simulink model "EKF_OPT"  (R2024b)
settings: Solver=FixedStepAuto  StartTime=0.0  StopTime=250  FixedStep=0.05  RelTol=1e-3
values from neighbouring files (symbols this model uses):
  D = diag(dvec)    [singleRun.m]
undefined symbols (not defined in the file or in its folder): DiscIntNeverNeededParam, IRED, mRED, P_ic, x_ic, x_rel
libraries: slpidlib x6, simulink x2
(part 1 of 2)
settings Model: Creator=ryang  LastModifiedBy=ryang

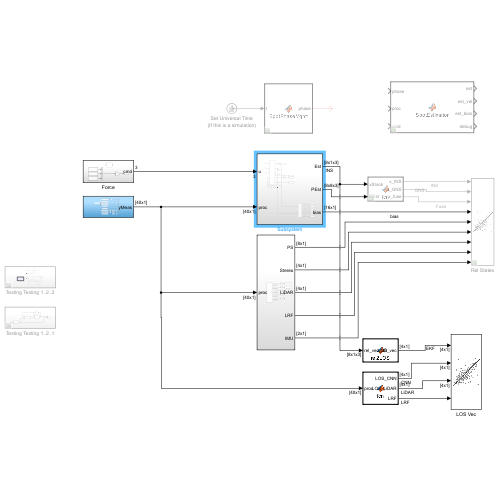
[thumbnail: Simulink's stored preview of the top-level diagram]
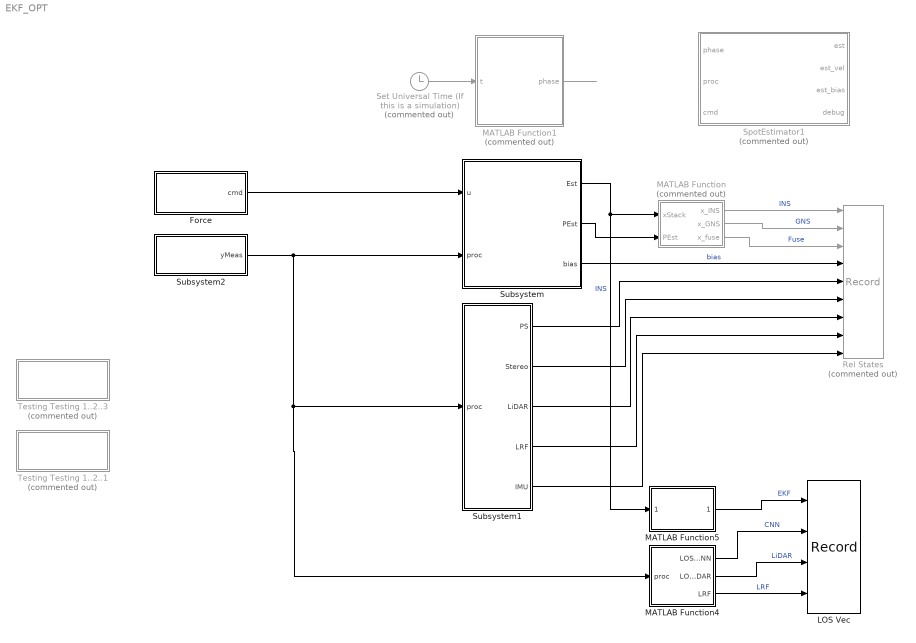
== system EKF_OPT ==
  Force : Subsystem
  LOS Vec : Record  FileSettingsInternal="{\"entries\":[{\"content\":{\"excelSettings\":{\"content\":{},\"type\":\"Streamout.ExcelSettings\"}},\"type\":\"Streamout.FileSettingStorage\",\"uuid\":\"\"}],\"packageUris\":[\"http:\\/\\/schema.mathworks.com\\/mf0\\/streamout_blocks\\/R2020a\"],\"version\":\"1.0\"}"  Layout=[2 2]  SignalsInternal="{\"entries\":[{\"content\":{\"signals\":[{\"content\":{\"blockPath\":[],\"dimensions\":[4,1],\"domain\":\"\",\"hasChildren\":true,\"lineColor\":\"#edb120\",\"lineWidth\":2,\"port\":1,\"sid\":[\"\"],\"signalID\":1,\"signalName\":\"EKF\"},\"type\":\"RecordBlkView.Signal\",\"uuid\":\"\"},{\"content\":{\"blockPath\":[],\"channel\":[1,1],\"dimensions\":[4,1],\"domain\":\"\",\"lineColor\":\"#139fff\",\"lineWidth\":2,\"parentID\":1,\"plots\":[ 1 ],\"port\":1,\"sid\":[\"\"],\"signalID\":2,\"signalName\":\"EKF\"},\"type\":\"RecordBlkView.Signal\",\"uuid\":\"\"},{\"content\":{\"blockPath\":[],\"dimensions\":[4,1],\"domain\":\"\",\"hasChildren\":true,\"lineColor\":\"#77ac30\",\"lineWidth\":2,\"port\":2,\"sid\":[\"\"],\"signalID\":3,\"signalName\":\"CNN\"},\"type\":\"RecordBlkView.Signal\",\"uuid\":\"\"},{\"content\":{\"blockPath\":[],\"channel\":[1,1],\"dimensions\":[4,1],\"domain\":\"\",\"lineColor\":\"#b746ff\",\"lineWidth\":2,\"parentID\":3,\"plots\":[ 1 ],\"port\":2,\"sid\":[\"\"],\"signalID\":4,\"signalName\":\"CNN\"},\"type\":\"RecordBlkView.Signal\",\"uuid\":\"\"},{\"content\":{\"blockPath\":[],\"dimensions\":[4,1],\"domain\":\"\",\"hasChildren\":true,\"lineColor\":\"#a2142f\",\"lineWidth\":2,\"port\":3,\"sid\":[\"\"],\"signalID\":5,\"signalName\":\"LiDAR\"},\"type\":\"RecordBlkView.Signal\",\"uuid\":\"\"},{\"content\":{\"blockPath\":[],\"channel\":[1,1],\"dimensions\":[4,1],\"domain\":\"\",\"lineColor\":\"#ff13a6\",\"lineWidth\":2,\"parentID\":5,\"plots\":[ 1 ],\"port\":3,\"sid\":[\"\"],\"signalID\":6,\"signalName\":\"LiDAR\"},\"type\":\"RecordBlkView.Signal\",\"uuid\":\"\"},{\"content\":{\"blockPath\":[],\"dimensions\":[1],\"domain\":\"\",\"lineColor\":\"#4dbeee\",\"lineWidth\":2,\"port\":4,\"sid\":[\"\"],\"signalID\":7,\"signalName\":\"LRF\"},\"type\":\"RecordBlkView.Signal\",\"uuid\":\"\"},{\"content\":{\"blockPath\":[],\"channel\":[2,1],\"dimensions\":[4,1],\"domain\":\"\",\"lineColor\":\"#fe330a\",\"lineWidth\":2,\"parentID\":1,\"plots\":[ 9 ],\"port\":1,\"sid\":[\"\"],\"signalID\":8,\"signalName\":\"EKF\"},\"type\":\"RecordBlkView.Signal\",\"uuid\":\"\"},{\"content\":{\"blockPath\":[],\"channel\":[3,1],\"dimensions\":[4,1],\"domain\":\"\",\"lineColor\":\"#22b573\",\"lineWidth\":2,\"parentID\":1,\"plots\":[ 2 ],\"port\":1,\"sid\":[\"\"],\"signalID\":9,\"signalName\":\"EKF\"},\"type\":\"RecordBlkView.Signal\",\"uuid\":\"\"},{\"content\":{\"blockPath\":[],\"channel\":[4,1],\"dimensions\":[4,1],\"domain\":\"\",\"lineColor\":\"#0072bd\",\"lineWidth\":2,\"parentID\":1,\"port\":1,\"sid\":[\"\"],\"signalID\":10,\"signalName\":\"EKF\"},\"type\":\"RecordBlkView.Signal\",\"uuid\":\"\"},{\"content\":{\"blockPath\":[],\"channel\":[2,1],\"dimensions\":[4,1],\"domain\":\"\",\"lineColor\":\"#d95319\",\"lineWidth\":2,\"parentID\":3,\"port\":2,\"sid\":[\"\"],\"signalID\":11,\"signalName\":\"CNN\"},\"type\":\"RecordBlkView.Signal\",\"uuid\":\"\"},{\"content\":{\"blockPath\":[],\"channel\":[3,1],\"dimensions\":[4,1],\"domain\":\"\",\"lineColor\":\"#edb120\",\"lineWidth\":2,\"parentID\":3,\"plots\":[ 2 ],\"port\":2,\"sid\":[\"\"],\"signalID\":12,\"signalName\":\"CNN\"},\"type\":\"RecordBlkView.Signal\",\"uuid\":\"\"},{\"content\":{\"blockPath\":[],\"channel\":[4,1],\"dimensions\":[4,1],\"domain\":\"\",\"lineColor\":\"#7e2f8e\",\"lineWidth\":2,\"parentID\":3,\"port\":2,\"sid\":[\"\"],\"signalID\":13,\"signalName\":\"CNN\"},\"type\":\"RecordBlkView.Signal\",\"uuid\":\"\"},{\"content\":{\"blockPath\":[],\"channel\":[2,1],\"dimensions\":[4,1],\"domain\":\"\",\"lineColor\":\"#77ac30\",\"lineWidth\":2,\"parentID\":5,\"plots\":[ 9 ],\"port\":3,\"sid\":[\"\"],\"signalID\":14,\"signalName\":\"LiDAR\"},\"type\":\"RecordBlkView.Signal\",\"uuid\":\"\"},{\"content\":{\"blockPath\":[],\"channel\":[3,1],\"dimensions\":[4,1],\"domain\":\"\",\"lineColor\":\"#4dbeee\",\"lineWidth\":2,\"parentID\":5,\"plots\":[ 2 ],\"port\":3,\"sid\":[\"\"],\"signalID\":15,\"signalName\":\"LiDAR\"},\"type\":\"RecordBlkView.Signal\",\"uuid\":\"\"},{\"content\":{\"blockPath\":[],\"channel\":[4,1],\"dimensions\":[4,1],\"domain\":\"\",\"lineColor\":\"#a2142f\",\"lineWidth\":2,\"parentID\":5,\"port\":3,\"sid\":[\"\"],\"signalID\":16,\"signalName\":\"LiDAR\"},\"type\":\"RecordBlkView.Signal\",\"uuid\":\"\"}]},\"type\":\"RecordBlkView.InputSignals\",\"uuid\":\"\"}],\"packageUris\":[\"http:\\/\\/schema.mathworks.com\\/mf0\\/streamout_blocks\\/R2020a\"],\"version\":\"1.0\"}"  CompatibilityTag=XY
  MATLAB Function : MATLAB Function  Commented=on  TreatAsAtomicUnit=on
  MATLAB Function1 : MATLAB Function  Commented=on  TreatAsAtomicUnit=on
  MATLAB Function4 : MATLAB Function  TreatAsAtomicUnit=on
  MATLAB Function5 : MATLAB Function  TreatAsAtomicUnit=on
  Rel States : Record  Commented=on  FileSettingsInternal="{\"entries\":[{\"content\":{\"excelSettings\":{\"content\":{},\"type\":\"Streamout.ExcelSettings\"}},\"type\":\"Streamout.FileSettingStorage\",\"uuid\":\"\"}],\"packageUris\":[\"http:\\/\\/schema.mathworks.com\\/mf0\\/streamout_blocks\\/R2020a\"],\"version\":\"1.0\"}"  Layout=[2 2]  SignalsInternal="{\"entries\":[{\"content\":{},\"type\":\"RecordBlkView.InputSignals\",\"uuid\":\"\"}],\"packageUris\":[\"http:\\/\\/schema.mathworks.com\\/mf0\\/streamout_blocks\\/R2020a\"],\"version\":\"1.0\"}"  CompatibilityTag=XY
  Set Universal Time (If this is a simulation) : Clock  Commented=on
  SpotEstimator1 : MATLAB Function  Commented=on  TreatAsAtomicUnit=on
  Subsystem : Subsystem
  Subsystem1 : Subsystem
  Subsystem2 : Subsystem
  Testing Testing 1..2..1 : Subsystem  Commented=on
  Testing Testing 1..2..3 : Subsystem  Commented=on
  wires:
  Set Universal Time (If this is a simulation)/1 -> MATLAB Function1/1(t)
  MATLAB Function1/1(phase) -> ?
  Subsystem2/1(yMeas) -> MATLAB Function4/1(proc), Subsystem1/1(proc), Subsystem/2(proc)
  MATLAB Function5/1(LOS_vec) -> LOS Vec/1  "EKF"
  MATLAB Function4/1(LOS_CNN) -> LOS Vec/2  "CNN"
  MATLAB Function4/2(LOS_LiDAR) -> LOS Vec/3  "LiDAR"
  MATLAB Function4/3(LRF) -> LOS Vec/4  "LRF"
  Subsystem/1(Est) -> MATLAB Function5/1(rel_vec_3D), MATLAB Function/1(xStack)  "INS"
  Force/1(cmd) -> Subsystem/1(u)
  MATLAB Function/1(x_INS) -> Rel States/1  "INS"
  MATLAB Function/2(x_GNS) -> Rel States/2  "GNS"
  MATLAB Function/3(x_fuse) -> Rel States/3  "Fuse"
  Subsystem/2(PEst) -> MATLAB Function/2(PEst)
  Subsystem/3(bias) -> Rel States/4  "bias"
  Subsystem1/1(PS) -> Rel States/5
  Subsystem1/2(Stereo) -> Rel States/6
  Subsystem1/3(LiDAR) -> Rel States/7
  Subsystem1/4(LRF) -> Rel States/8
  Subsystem1/5(IMU) -> Rel States/9

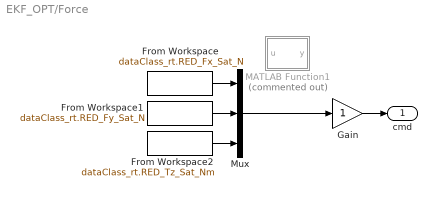
== system EKF_OPT/Force ==
  From Workspace : FromWorkspace  VariableName=dataClass_rt.RED_Fx_Sat_N
  From Workspace1 : FromWorkspace  VariableName=dataClass_rt.RED_Fy_Sat_N
  From Workspace2 : FromWorkspace  VariableName=dataClass_rt.RED_Tz_Sat_Nm
  Gain : Gain
  MATLAB Function1 : MATLAB Function  Commented=on  TreatAsAtomicUnit=on
  Mux : Mux  Inputs=3
  cmd : Outport
  wires:
  From Workspace2/1 -> Mux/3
  From Workspace1/1 -> Mux/2
  From Workspace/1 -> Mux/1
  Gain/1 -> cmd/1
  Mux/1 -> Gain/1

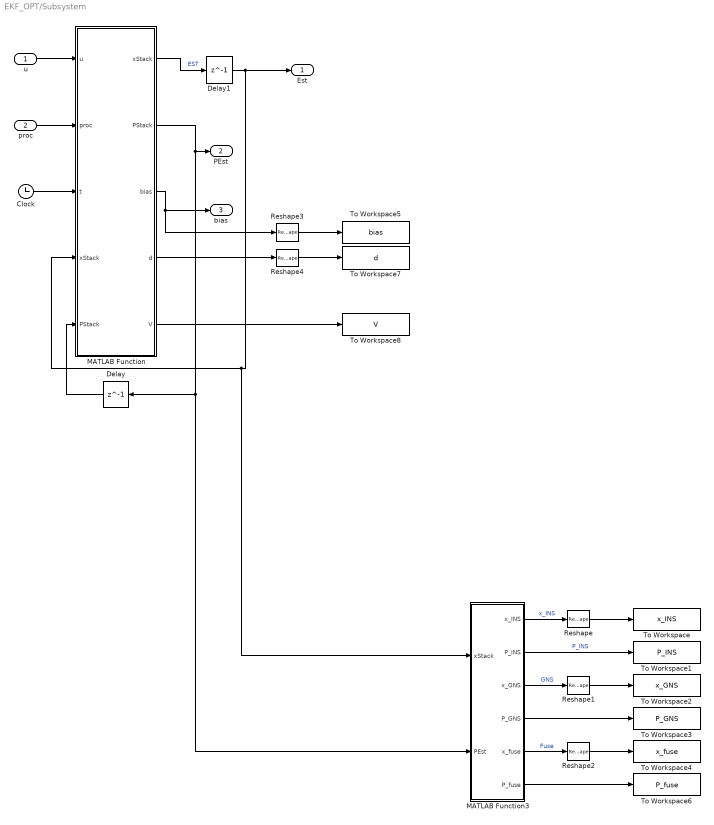
== system EKF_OPT/Subsystem ==
  u : Inport
  proc : Inport  Port=2
  Clock : Clock
  Delay : Delay  DelayLength=1  InitialCondition=P_ic
  Delay1 : Delay  DelayLength=1  InitialCondition=x_ic
  MATLAB Function : MATLAB Function  TreatAsAtomicUnit=on
  MATLAB Function3 : MATLAB Function  TreatAsAtomicUnit=on
  Reshape{,1..4} (5 alike) : Reshape  OutputDimensionality=Row vector (2-D)
  To Workspace : ToWorkspace  VariableName=x_INS  SampleTime=-1
      settings: Save2DSignal=2-D array (concatenate along first dimension)
  To Workspace1 : ToWorkspace  VariableName=P_INS  SampleTime=-1
  To Workspace2 : ToWorkspace  VariableName=x_GNS  SampleTime=-1
      settings: Save2DSignal=2-D array (concatenate along first dimension)
  To Workspace3 : ToWorkspace  VariableName=P_GNS  SampleTime=-1
  To Workspace4 : ToWorkspace  VariableName=x_fuse  SampleTime=-1
      settings: Save2DSignal=2-D array (concatenate along first dimension)
  To Workspace5 : ToWorkspace  VariableName=bias  SampleTime=-1
      settings: Save2DSignal=2-D array (concatenate along first dimension)
  To Workspace6 : ToWorkspace  VariableName=P_fuse  SampleTime=-1
  To Workspace7 : ToWorkspace  VariableName=d  SampleTime=-1
      settings: Save2DSignal=2-D array (concatenate along first dimension)
  To Workspace8 : ToWorkspace  VariableName=V  SampleTime=-1
  Est : Outport
  PEst : Outport  Port=2
  bias : Outport  Port=3
  wires:
  proc/1 -> MATLAB Function/2(proc)
  u/1 -> MATLAB Function/1(u)
  MATLAB Function/1(xStack) -> Delay1/1  "EST"
  Delay/1 -> MATLAB Function/5("PStack ")
  MATLAB Function/2(PStack) -> MATLAB Function3/2(PEst), Delay/1, PEst/1
  Delay1/1 -> MATLAB Function3/1(xStack), MATLAB Function/4("xStack "), Est/1
  MATLAB Function/3(bias) -> Reshape3/1, bias/1
  Clock/1 -> MATLAB Function/3(t)
  MATLAB Function3/2(P_INS) -> To Workspace1/1  "P_INS"
  MATLAB Function3/3(x_GNS) -> Reshape1/1  "GNS"
  MATLAB Function3/4(P_GNS) -> To Workspace3/1
  MATLAB Function3/5(x_fuse) -> Reshape2/1  "Fuse"
  MATLAB Function3/6(P_fuse) -> To Workspace6/1
  MATLAB Function3/1(x_INS) -> Reshape/1  "x_INS"
  Reshape/1 -> To Workspace/1
  Reshape1/1 -> To Workspace2/1
  Reshape2/1 -> To Workspace4/1
  Reshape3/1 -> To Workspace5/1
  MATLAB Function/4(d) -> Reshape4/1
  Reshape4/1 -> To Workspace7/1
  MATLAB Function/5(V) -> To Workspace8/1

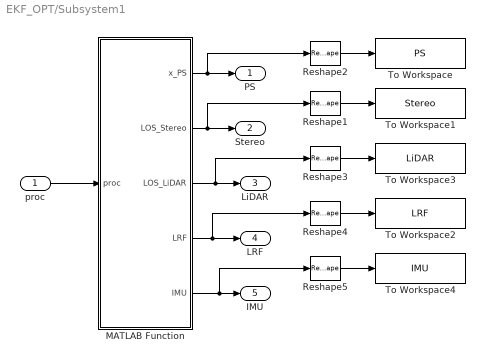
== system EKF_OPT/Subsystem1 ==
  proc : Inport
  MATLAB Function : MATLAB Function  TreatAsAtomicUnit=on
  Reshape{1..5} (5 alike) : Reshape  OutputDimensionality=Row vector (2-D)
  To Workspace : ToWorkspace  VariableName=PS  SampleTime=-1
      settings: Save2DSignal=2-D array (concatenate along first dimension)
  To Workspace1 : ToWorkspace  VariableName=Stereo  SampleTime=-1
      settings: Save2DSignal=2-D array (concatenate along first dimension)
  To Workspace2 : ToWorkspace  VariableName=LRF  SampleTime=-1
      settings: Save2DSignal=2-D array (concatenate along first dimension)
  To Workspace3 : ToWorkspace  VariableName=LiDAR  SampleTime=-1
      settings: Save2DSignal=2-D array (concatenate along first dimension)
  To Workspace4 : ToWorkspace  VariableName=IMU  SampleTime=-1
      settings: Save2DSignal=2-D array (concatenate along first dimension)
  PS : Outport
  Stereo : Outport  Port=2
  LiDAR : Outport  Port=3
  LRF : Outport  Port=4
  IMU : Outport  Port=5
  wires:
  proc/1 -> MATLAB Function/1(proc)
  MATLAB Function/1(x_PS) -> Reshape2/1, PS/1
  MATLAB Function/2(LOS_Stereo) -> Reshape1/1, Stereo/1
  MATLAB Function/3(LOS_LiDAR) -> Reshape3/1, LiDAR/1
  MATLAB Function/5(IMU) -> Reshape5/1, IMU/1
  MATLAB Function/4(LRF) -> Reshape4/1, LRF/1
  Reshape2/1 -> To Workspace/1
  Reshape1/1 -> To Workspace1/1
  Reshape3/1 -> To Workspace3/1
  Reshape4/1 -> To Workspace2/1
  Reshape5/1 -> To Workspace4/1

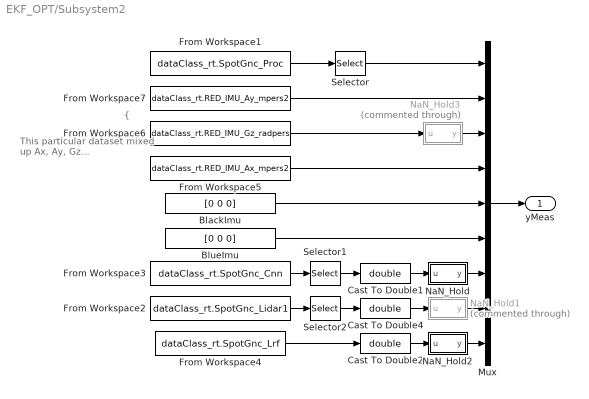
== system EKF_OPT/Subsystem2 ==
  note: {
  note: This particular dataset
      | mixed up Ax, Ay, Gz...
  BlackImu : Constant  Value=[0 0 0]
  BlueImu : Constant  Value=[0 0 0]
  Cast To Double1 : DataTypeConversion  OutDataTypeStr=double  SaturateOnIntegerOverflow=off  RndMeth=Floor
  Cast To Double2 : DataTypeConversion  OutDataTypeStr=double  SaturateOnIntegerOverflow=off  RndMeth=Floor
  Cast To Double4 : DataTypeConversion  OutDataTypeStr=double  SaturateOnIntegerOverflow=off  RndMeth=Floor
  From Workspace1 : FromWorkspace  VariableName=dataClass_rt.SpotGnc_Proc
  From Workspace2 : FromWorkspace  VariableName=dataClass_rt.SpotGnc_Lidar1
  From Workspace3 : FromWorkspace  VariableName=dataClass_rt.SpotGnc_Cnn
  From Workspace4 : FromWorkspace  VariableName=dataClass_rt.SpotGnc_Lrf
  From Workspace5 : FromWorkspace  VariableName=dataClass_rt.RED_IMU_Ax_mpers2
  From Workspace6 : FromWorkspace  VariableName=dataClass_rt.RED_IMU_Gz_radpers
  From Workspace7 : FromWorkspace  VariableName=dataClass_rt.RED_IMU_Ay_mpers2
  Mux : Mux  Inputs=9
  NaN_Hold : Subsystem
  NaN_Hold1 : Subsystem  Commented=through
  NaN_Hold2 : Subsystem
  NaN_Hold3 : Subsystem  Commented=through
  Selector : Selector  InputPortWidth=40  IndexOptions=Index vector (dialog)  Indices=[1:24]  OutputSizes=1
  Selector1 : Selector  InputPortWidth=4  IndexOptions=Index vector (dialog)  Indices=[1 2 3]  OutputSizes=1
  Selector2 : Selector  InputPortWidth=5  IndexOptions=Index vector (dialog)  Indices=[1 2 3]  OutputSizes=1
  yMeas : Outport
  wires:
  Selector/1 -> Mux/1
  Mux/1 -> yMeas/1
  From Workspace1/1 -> Selector/1
  Selector2/1 -> Cast To Double4/1
  Selector1/1 -> Cast To Double1/1
  Cast To Double1/1 -> NaN_Hold/1(u)
  From Workspace4/1 -> Cast To Double2/1
  BlackImu/1 -> Mux/5
  From Workspace2/1 -> Selector2/1
  BlueImu/1 -> Mux/6
  Cast To Double4/1 -> NaN_Hold1/1(u)
  From Workspace5/1 -> Mux/4
  From Workspace6/1 -> NaN_Hold3/1(u)
  From Workspace7/1 -> Mux/2
  Cast To Double2/1 -> NaN_Hold2/1(u)
  From Workspace3/1 -> Selector1/1
  NaN_Hold/1(y) -> Mux/7
  NaN_Hold1/1(y) -> Mux/8
  NaN_Hold2/1(y) -> Mux/9
  NaN_Hold3/1(y) -> Mux/3

== system EKF_OPT/Testing Testing 1..2..1 ==
  Clock : Clock
  Delay2 : Delay  DelayLength=1  InitialCondition=x_rel
  LQR+FeedForward : Subsystem
  MATLAB Function : MATLAB Function  TreatAsAtomicUnit=on
  MATLAB Function3 : MATLAB Function  TreatAsAtomicUnit=on
  XY Graph : Record  FileSettingsInternal="{\"entries\":[{\"content\":{\"excelSettings\":{\"content\":{},\"type\":\"Streamout.ExcelSettings\"}},\"type\":\"Streamout.FileSettingStorage\",\"uuid\":\"\"}],\"packageUris\":[\"http:\\/\\/schema.mathworks.com\\/mf0\\/streamout_blocks\\/R2020a\"],\"version\":\"1.0\"}"  Layout=[2 2]  SignalsInternal="{\"entries\":[{\"content\":{\"signals\":[{\"content\":{\"blockPath\":[],\"dimensions\":[8,1],\"domain\":\"\",\"hasChildren\":true,\"lineColor\":\"#fe330a\",\"lineWidth\":2,\"port\":1,\"signalID\":1,\"signalName\":\"true\"},\"type\":\"RecordBlkView.Signal\",\"uuid\":\"\"},{\"content\":{\"blockPath\":[],\"channel\":[1,1],\"dimensions\":[8,1],\"domain\":\"\",\"lineColor\":\"#a2142f\",\"lineWidth\":2,\"parentID\":1,\"plots\":[ 1 ],\"port\":1,\"signalID\":2,\"signalName\":\"true\"},\"type\":\"RecordBlkView.Signal\",\"uuid\":\"\"},{\"content\":{\"blockPath\":[],\"channel\":[2,1],\"dimensions\":[8,1],\"domain\":\"\",\"lineColor\":\"#0072bd\",\"lineWidth\":2,\"parentID\":1,\"plots\":[ 9 ],\"port\":1,\"signalID\":3,\"signalName\":\"true\"},\"type\":\"RecordBlkView.Signal\",\"uuid\":\"\"},{\"content\":{\"blockPath\":[],\"channel\":[3,1],\"dimensions\":[8,1],\"domain\":\"\",\"lineColor\":\"#d95319\",\"lineWidth\":2,\"parentID\":1,\"port\":1,\"signalID\":4,\"signalName\":\"true\"},\"type\":\"RecordBlkView.Signal\",\"uuid\":\"\"},{\"content\":{\"blockPath\":[],\"channel\":[4,1],\"dimensions\":[8,1],\"domain\":\"\",\"lineColor\":\"#edb120\",\"lineWidth\":2,\"parentID\":1,\"port\":1,\"signalID\":5,\"signalName\":\"true\"},\"type\":\"RecordBlkView.Signal\",\"uuid\":\"\"},{\"content\":{\"blockPath\":[],\"channel\":[5,1],\"dimensions\":[8,1],\"domain\":\"\",\"lineColor\":\"#7e2f8e\",\"lineWidth\":2,\"parentID\":1,\"port\":1,\"signalID\":6,\"signalName\":\"true\"},\"type\":\"RecordBlkView.Signal\",\"uuid\":\"\"},{\"content\":{\"blockPath\":[],\"channel\":[6,1],\"dimensions\":[8,1],\"domain\":\"\",\"lineColor\":\"#77ac30\",\"lineWidth\":2,\"parentID\":1,\"port\":1,\"signalID\":7,\"signalName\":\"true\"},\"type\":\"RecordBlkView.Signal\",\"uuid\":\"\"},{\"content\":{\"blockPath\":[],\"channel\":[7,1],\"dimensions\":[8,1],\"domain\":\"\",\"lineColor\":\"#4dbeee\",\"lineWidth\":2,\"parentID\":1,\"plots\":[ 2 ],\"port\":1,\"signalID\":8,\"signalName\":\"true\"},\"type\":\"RecordBlkView.Signal\",\"uuid\":\"\"},{\"content\":{\"blockPath\":[],\"channel\":[8,1],\"dimensions\":[8,1],\"domain\":\"\",\"lineColor\":\"#a2142f\",\"lineWidth\":2,\"parentID\":1,\"plots\":[ 10 ],\"port\":1,\"signalID\":9,\"signalName\":\"true\"},\"type\":\"RecordBlkView.Signal\",\"uuid\":\"\"},{\"content\":{\"blockPath\":[],\"dimensions\":[6,1],\"domain\":\"\",\"hasChildren\":true,\"lineColor\":\"#0072bd\",\"lineWidth\":2,\"port\":2,\"signalID\":10,\"signalName\":\"Ref\"},\"type\":\"RecordBlkView.Signal\",\"uuid\":\"\"},{\"content\":{\"blockPath\":[],\"channel\":[1,1],\"dimensions\":[6,1],\"domain\":\"\",\"lineColor\":\"#ff6929\",\"lineWidth\":2,\"parentID\":10,\"plots\":[ 1 ],\"port\":2,\"signalID\":11,\"signalName\":\"Ref\"},\"type\":\"RecordBlkView.Signal\",\"uuid\":\"\"},{\"content\":{\"blockPath\":[],\"channel\":[2,1],\"dimensions\":[6,1],\"domain\":\"\",\"lineColor\":\"#b746ff\",\"lineWidth\":2,\"parentID\":10,\"plots\":[ 9 ],\"port\":2,\"signalID\":12,\"signalName\":\"Ref\"},\"type\":\"RecordBlkView.Signal\",\"uuid\":\"\"},{\"content\":{\"blockPath\":[],\"channel\":[3,1],\"dimensions\":[6,1],\"domain\":\"\",\"lineColor\":\"#64d413\",\"lineWidth\":2,\"parentID\":10,\"plots\":[ 2 ],\"port\":2,\"signalID\":13,\"signalName\":\"Ref\"},\"type\":\"RecordBlkView.Signal\",\"uuid\":\"\"},{\"content\":{\"blockPath\":[],\"channel\":[4,1],\"dimensions\":[6,1],\"domain\":\"\",\"lineColor\":\"#ff13a6\",\"lineWidth\":2,\"parentID\":10,\"port\":2,\"signalID\":14,\"signalName\":\"Ref\"},\"type\":\"RecordBlkView.Signal\",\"uuid\":\"\"},{\"content\":{\"blockPath\":[],\"channel\":[5,1],\"dimensions\":[6,1],\"domain\":\"\",\"lineColor\":\"#fe330a\",\"lineWidth\":2,\"parentID\":10,\"port\":2,\"signalID\":15,\"signalName\":\"Ref\"},\"type\":\"RecordBlkView.Signal\",\"uuid\":\"\"},{\"content\":{\"blockPath\":[],\"channel\":[6,1],\"dimensions\":[6,1],\"domain\":\"\",\"lineColor\":\"#22b573\",\"lineWidth\":2,\"parentID\":10,\"port\":2,\"signalID\":16,\"signalName\":\"Ref\"},\"type\":\"RecordBlkView.Signal\",\"uuid\":\"\"}]},\"type\":\"RecordBlkView.InputSignals\",\"uuid\":\"\"}],\"packageUris\":[\"http:\\/\\/schema.mathworks.com\\/mf0\\/streamout_blocks\\/R2020a\"],\"version\":\"1.0\"}"  CompatibilityTag=XY
  wires:
  MATLAB Function3/1(x_new) -> XY Graph/1, Delay2/1  "true"
  Delay2/1 -> LQR+FeedForward/1(true), MATLAB Function3/1(x_old)
  MATLAB Function/1(ref_traj) -> LQR+FeedForward/2(ref_traj), XY Graph/2  "Ref"
  Clock/1 -> MATLAB Function/1(t)
  LQR+FeedForward/1(u) -> MATLAB Function3/2(u)

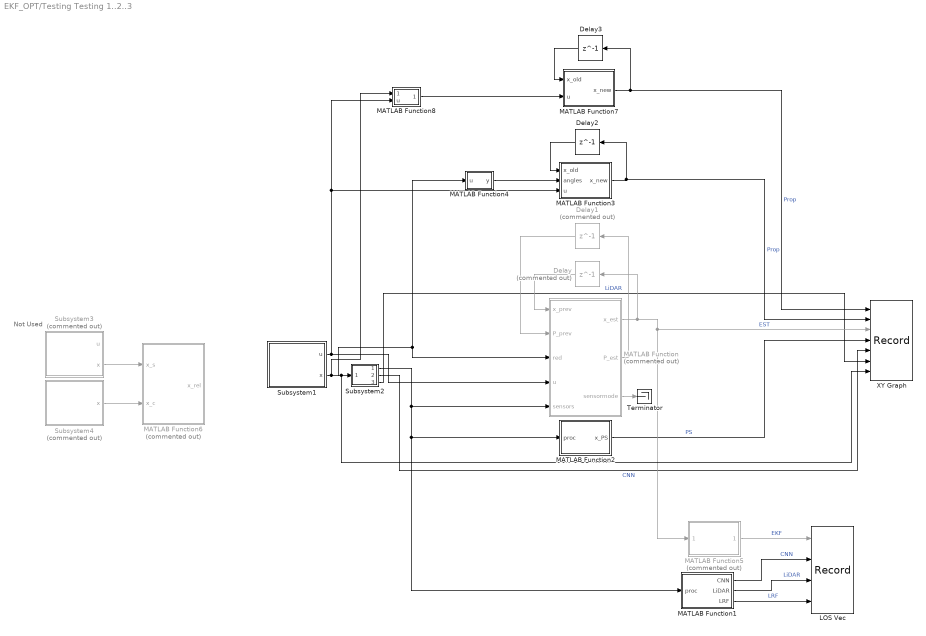
== system EKF_OPT/Testing Testing 1..2..3 ==
  note: Not Used
  Delay : Delay  Commented=on  DelayLength=1  InitialCondition=x_rel
  Delay1 : Delay  Commented=on  DelayLength=1  InitialCondition=0.2*eye(6)
  Delay2 : Delay  DelayLength=1  InitialCondition=x_rel(1:6)
  Delay3 : Delay  DelayLength=1  InitialCondition=x_rel
  LOS Vec : Record  FileSettingsInternal="{\"entries\":[{\"content\":{\"excelSettings\":{\"content\":{},\"type\":\"Streamout.ExcelSettings\"}},\"type\":\"Streamout.FileSettingStorage\",\"uuid\":\"\"}],\"packageUris\":[\"http:\\/\\/schema.mathworks.com\\/mf0\\/streamout_blocks\\/R2020a\"],\"version\":\"1.0\"}"  Layout=[1 1]  SignalsInternal="{\"entries\":[{\"content\":{},\"type\":\"RecordBlkView.InputSignals\",\"uuid\":\"\"}],\"packageUris\":[\"http:\\/\\/schema.mathworks.com\\/mf0\\/streamout_blocks\\/R2020a\"],\"version\":\"1.0\"}"  VisualizationBindings="{\"sparklinesplugin\":{\"info\":[{\"bindingParametersList\":[],\"subplotID\":1}]}}"  CompatibilityTag=XY
  MATLAB Function : MATLAB Function  Commented=on  TreatAsAtomicUnit=on
  MATLAB Function1 : MATLAB Function  TreatAsAtomicUnit=on
  MATLAB Function2 : MATLAB Function  TreatAsAtomicUnit=on
  MATLAB Function3 : MATLAB Function  TreatAsAtomicUnit=on
  MATLAB Function4 : MATLAB Function  TreatAsAtomicUnit=on
  MATLAB Function5 : MATLAB Function  Commented=on  TreatAsAtomicUnit=on
  MATLAB Function6 : MATLAB Function  Commented=on  TreatAsAtomicUnit=on
  MATLAB Function7 : MATLAB Function  TreatAsAtomicUnit=on
  MATLAB Function8 : MATLAB Function  TreatAsAtomicUnit=on
  Subsystem1 : Subsystem
  Subsystem2 : Subsystem
  Subsystem3 : Subsystem  Commented=on
  Subsystem4 : Subsystem  Commented=on
  Terminator : Terminator
  XY Graph : Record  FileSettingsInternal="{\"entries\":[{\"content\":{\"excelSettings\":{\"content\":{},\"type\":\"Streamout.ExcelSettings\"}},\"type\":\"Streamout.FileSettingStorage\",\"uuid\":\"\"}],\"packageUris\":[\"http:\\/\\/schema.mathworks.com\\/mf0\\/streamout_blocks\\/R2020a\"],\"version\":\"1.0\"}"  Layout=[2 2]  SignalsInternal="{\"entries\":[{\"content\":{},\"type\":\"RecordBlkView.InputSignals\",\"uuid\":\"\"}],\"packageUris\":[\"http:\\/\\/schema.mathworks.com\\/mf0\\/streamout_blocks\\/R2020a\"],\"version\":\"1.0\"}"  CompatibilityTag=XY
  wires:
  MATLAB Function1/1(CNN) -> LOS Vec/2  "CNN"
  Subsystem2/3(LiDAR) -> XY Graph/6  "LiDAR"
  MATLAB Function5/1(LOS_vec) -> LOS Vec/1  "EKF"
  Subsystem2/2(CNN) -> XY Graph/5  "CNN"
  MATLAB Function1/2(LiDAR) -> LOS Vec/3  "LiDAR"
  MATLAB Function2/1(x_PS) -> XY Graph/4  "PS"
  MATLAB Function/3(sensormode) -> Terminator/1
  MATLAB Function/2(P_est) -> Delay1/1
  Subsystem2/1(proc) -> MATLAB Function1/1(proc), MATLAB Function2/1(proc), MATLAB Function/5(sensors)
  Delay/1 -> MATLAB Function/1(x_prev)
  Delay1/1 -> MATLAB Function/2(P_prev)
  MATLAB Function1/3(LRF) -> LOS Vec/4  "LRF"
  MATLAB Function/1(x_est) -> Delay/1, MATLAB Function5/1(rel_vec), XY Graph/3  "EST"
  Subsystem1/1(u) -> MATLAB Function8/2(u), MATLAB Function3/3(u), MATLAB Function/4(u)
  Subsystem1/2(x) -> MATLAB Function8/1(theta), MATLAB Function4/1(u), MATLAB Function/3(red), XY Graph/7, Subsystem2/1(RED)
  MATLAB Function3/1(x_new) -> XY Graph/2, Delay2/1  "Prop"
  Delay2/1 -> MATLAB Function3/1(x_old)
  MATLAB Function4/1(y) -> MATLAB Function3/2(angles)
  Subsystem3/2(x) -> MATLAB Function6/1(x_s)
  Subsystem4/1(x) -> MATLAB Function6/2(x_c)
  MATLAB Function7/1(x_new) -> XY Graph/1, Delay3/1  "Prop"
  Delay3/1 -> MATLAB Function7/1(x_old)
  MATLAB Function8/1(u_body) -> MATLAB Function7/2(u)

== system EKF_OPT/Subsystem2/NaN_Hold ==
  u : Inport
  Delay : Delay  DelayLength=1
  MATLAB Function : MATLAB Function  TreatAsAtomicUnit=on
  y : Outport
  wires:
  u/1 -> Delay/1, MATLAB Function/1(u_curr)
  MATLAB Function/1(y) -> y/1
  Delay/1 -> MATLAB Function/2(u_prev)

== system EKF_OPT/Subsystem2/NaN_Hold1 ==
  u : Inport
  Delay : Delay  DelayLength=1
  MATLAB Function : MATLAB Function  TreatAsAtomicUnit=on
  y : Outport
  wires:
  u/1 -> Delay/1, MATLAB Function/1(u_curr)
  MATLAB Function/1(y) -> y/1
  Delay/1 -> MATLAB Function/2(u_prev)

== system EKF_OPT/Subsystem2/NaN_Hold2 ==
  u : Inport
  Delay : Delay  DelayLength=1
  MATLAB Function : MATLAB Function  TreatAsAtomicUnit=on
  y : Outport
  wires:
  u/1 -> Delay/1, MATLAB Function/1(u_curr)
  MATLAB Function/1(y) -> y/1
  Delay/1 -> MATLAB Function/2(u_prev)

== system EKF_OPT/Subsystem2/NaN_Hold3 ==
  u : Inport
  Delay : Delay  DelayLength=1
  MATLAB Function : MATLAB Function  TreatAsAtomicUnit=on
  y : Outport
  wires:
  Delay/1 -> MATLAB Function/2(u_prev)
  MATLAB Function/1(y) -> y/1
  u/1 -> MATLAB Function/1(u_curr), Delay/1

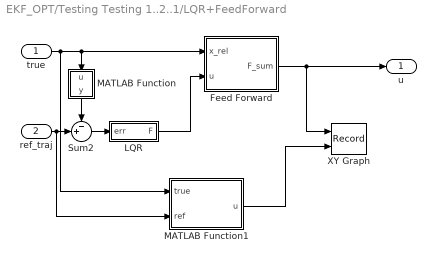
== system EKF_OPT/Testing Testing 1..2..1/LQR+FeedForward ==
  true : Inport
  ref_traj : Inport  Port=2
  Feed Forward : MATLAB Function  TreatAsAtomicUnit=on
  LQR : MATLAB Function  TreatAsAtomicUnit=on
  MATLAB Function : MATLAB Function  TreatAsAtomicUnit=on
  MATLAB Function1 : MATLAB Function  TreatAsAtomicUnit=on
  Sum2 : Sum  Inputs=-+|
  XY Graph : Record  FileSettingsInternal="{\"entries\":[{\"content\":{\"excelSettings\":{\"content\":{},\"type\":\"Streamout.ExcelSettings\"}},\"type\":\"Streamout.FileSettingStorage\",\"uuid\":\"\"}],\"packageUris\":[\"http:\\/\\/schema.mathworks.com\\/mf0\\/streamout_blocks\\/R2020a\"],\"version\":\"1.0\"}"  Layout=[1 1]  SignalsInternal="{\"entries\":[{\"content\":{\"signals\":[{\"content\":{\"blockPath\":[],\"dimensions\":[1],\"domain\":\"\",\"lineColor\":\"#a2142f\",\"plots\":[ 1 ],\"port\":1,\"signalID\":1,\"signalName\":\"XY Graph:1\"},\"type\":\"RecordBlkView.Signal\",\"uuid\":\"\"},{\"content\":{\"blockPath\":[],\"dimensions\":[1],\"domain\":\"\",\"lineColor\":\"#139fff\",\"plots\":[ 1 ],\"port\":2,\"signalID\":2,\"signalName\":\"XY Graph:2\"},\"type\":\"RecordBlkView.Signal\",\"uuid\":\"\"}]},\"type\":\"RecordBlkView.InputSignals\",\"uuid\":\"\"}],\"packageUris\":[\"http:\\/\\/schema.mathworks.com\\/mf0\\/streamout_blocks\\/R2020a\"],\"version\":\"1.0\"}"  VisualizationBindings="{\"xyplotplugin\":{\"info\":[{\"series\":[{\"bindingParametersList\":[{\"parameter\":\"X-Axis\",\"signalID\":1,\"signalName\":\"XY Graph:1\"},{\"parameter\":\"Y-Axis\",\"signalID\":2,\"signalName\":\"XY Graph:2\"}],\"seriesID\":0}],\"subplotID\":1}]}}"  CompatibilityTag=XY
  u : Outport
  wires:
  Sum2/1 -> LQR/1(err)
  true/1 -> MATLAB Function1/1(true), MATLAB Function/1(u), Feed Forward/1(x_rel)
  ref_traj/1 -> MATLAB Function1/2(ref), Sum2/2
  MATLAB Function/1(y) -> Sum2/1
  LQR/1(F) -> Feed Forward/2(u)
  Feed Forward/1(F_sum) -> XY Graph/1, u/1
  MATLAB Function1/1(u) -> XY Graph/2

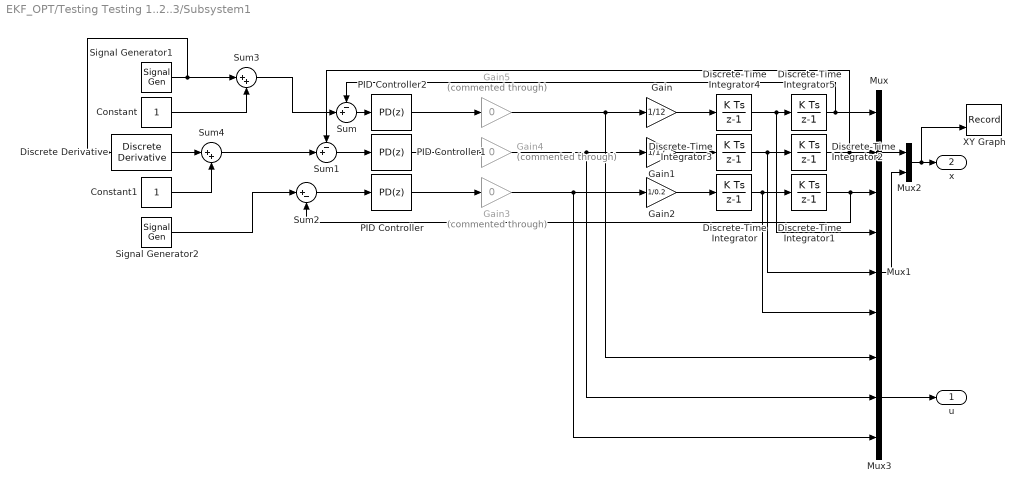
== system EKF_OPT/Testing Testing 1..2..3/Subsystem1 ==
  Constant : Constant
  Constant1 : Constant
  Discrete Derivative : simulink/Discrete/Discrete Derivative  gainval=1.0  ICPrevScaledInput=0.0  OutMin=[]  OutMax=[]  OutDataType=fixdt(1, 16)  OutScaling=2^-10  DoSatur=off
  Discrete-Time Integrator : DiscreteIntegrator  InitialCondition=-0.3  SampleTime=-1  ICPrevOutput=DiscIntNeverNeededParam  ICPrevScaledInput=DiscIntNeverNeededParam
  Discrete-Time Integrator1 : DiscreteIntegrator  SampleTime=-1  ICPrevOutput=DiscIntNeverNeededParam  ICPrevScaledInput=DiscIntNeverNeededParam
  Discrete-Time Integrator2 : DiscreteIntegrator  InitialCondition=2  SampleTime=-1  ICPrevOutput=DiscIntNeverNeededParam  ICPrevScaledInput=DiscIntNeverNeededParam
  Discrete-Time Integrator3 : DiscreteIntegrator  InitialCondition=0.2  SampleTime=-1  ICPrevOutput=DiscIntNeverNeededParam  ICPrevScaledInput=DiscIntNeverNeededParam
  Discrete-Time Integrator4 : DiscreteIntegrator  InitialCondition=-0.1  SampleTime=-1  ICPrevOutput=DiscIntNeverNeededParam  ICPrevScaledInput=DiscIntNeverNeededParam
  Discrete-Time Integrator5 : DiscreteIntegrator  InitialCondition=1  SampleTime=-1  ICPrevOutput=DiscIntNeverNeededParam  ICPrevScaledInput=DiscIntNeverNeededParam
  Gain : Gain  Gain=1/12
  Gain1 : Gain  Gain=1/12
  Gain2 : Gain  Gain=1/0.2
  Gain3 : Gain  Commented=through  Gain=0
  Gain4 : Gain  Commented=through  Gain=0
  Gain5 : Gain  Commented=through  Gain=0
  Mux : Mux  Inputs=3
  Mux1 : Mux  Inputs=3
  Mux2 : Mux  Inputs=2
  Mux3 : Mux  Inputs=3
  PID Controller : slpidlib/PID Controller  Controller=PD  Form=Parallel  TimeDomain=Discrete-time  UseExternalTs=off  SampleTime=-1  IntegratorMethod=Forward Euler  FilterMethod=Forward Euler  ControllerParametersSource=internal  P=0.00863228174020387  I=1  UseKiTs=off  D=0.441408383064275  UseExternalDerivativeSource=off  N=18.5475442531041  UseFilter=on  TunerSelectOption=Transfer Function Based (PID Tuner App)  InitialConditionSource=internal  InitialConditionForIntegrator=0  InitialConditionForFilter=0  DifferentiatorICPrevScaledInput=0  ExternalReset=none  TrackingMode=off  Kt=1  LimitOutput=off  SatLimitsSource=internal  UpperSaturationLimit=inf  LowerSaturationLimit=-inf  LinearizeAsGain=on  AntiWindupMode=none  Kb=1  LimitIntegrator=off  UpperIntegratorSaturationLimit=inf  LowerIntegratorSaturationLimit=-inf  POutMin=[]  POutMax=[]  IOutMin=[]  IOutMax=[]  DOutMin=[]  DOutMax=[]  NOutMin=[]  NOutMax=[]  SumOutMin=[]  SumOutMax=[]  SaturationOutMin=[]  SaturationOutMax=[]  PParamMin=[]  PParamMax=[]  IParamMin=[]  IParamMax=[]  DParamMin=[]  DParamMax=[]  NParamMin=[]  NParamMax=[]  KbParamMin=[]  KbParamMax=[]  KtParamMin=[]  KtParamMax=[]  KbOutMin=[]  KbOutMax=[]  KtOutMin=[]  KtOutMax=[]  IntegratorOutMin=[]  IntegratorOutMax=[]  FilterOutMin=[]  FilterOutMax=[]  SumI1OutMin=[]  SumI1OutMax=[]  SumI2OutMin=[]  SumI2OutMax=[]  SumI3OutMin=[]  SumI3OutMax=[]  SumI4OutMin=[]  SumI4OutMax=[]  SumDOutMin=[]  SumDOutMax=[]  DifferentiatorOutMin=[]  DifferentiatorOutMax=[]  FilterDiffOutCoefMin=[]  FilterDiffOutCoefMax=[]  ReciprocalOutMin=[]  ReciprocalOutMax=[]  SumDenOutMin=[]  SumDenOutMax=[]  SumNumOutMin=[]  SumNumOutMax=[]  DivideOutMin=[]  DivideOutMax=[]  UdiffTsProdOutMin=[]  UdiffTsProdOutMax=[]  NTsProdOutMin=[]  NTsProdOutMax=[]  UintegralTsProdOutMin=[]  UintegralTsProdOutMax=[]  UngainTsProdOutMin=[]  UngainTsProdOutMax=[]  ClampingZeroOutDataTypeStr=Inherit: Inherit via back propagation  ClampingZeroOutMin=[]  ClampingZeroOutMax=[]  FilterDenConstantOutDataTypeStr=Inherit: Inherit via back propagation  FilterDenConstantOutMin=[]  FilterDenConstantOutMax=[]  PCopyOutDataTypeStr=Inherit: Inherit via back propagation  PCopyOutMin=[]  PCopyOutMax=[]  NCopyOutDataTypeStr=Inherit: Inherit via back propagation  NCopyOutMin=[]  NCopyOutMax=[]  IntegratorContinuousStateAttributes=''  IntegratorStateMustResolveToSignalObject=off  IntegratorRTWStateStorageClass=Auto  FilterContinuousStateAttributes=''  FilterStateMustResolveToSignalObject=off  FilterRTWStateStorageClass=Auto  ParallelPVariant=InternalParameters  IdealPVariant=Disabled  IVariant=Disabled  DVariant=InternalParameters  IntegratorVariant=Disabled  SatVariant=Disabled  AWVariant=Disabled  PCopyVariant=Disabled  TRVariant=Disabled  FdbkBlocksVariant=Forward  IdealPFdbkVariant=Disabled  SatFdbkVariant=Disabled  DerivativeFilterVariant=ForwardEulerFilter  NVariant=InternalParameters  NCopyVariant=Disabled  FilterICVariant=InternalICsFilter  IntegratorICVariant=Disabled  ExternalResetVariant=Disabled  TRSumVariant=Passthrough  SumFdbkVariant=Disabled  SumVariant=Sum_PD  TsampFilterVariant=InternalTs  TsampNgainVariant=Passthrough  TsampIntegralVariant=Disabled_SignalSpec  ExternalSaturationOutDataTypeStr=Inherit: Same as second input  DerivativeSourceVariant=ErrorSignal  PreIntVariant=InternalPreInt
  PID Controller1 : slpidlib/PID Controller  Controller=PD  Form=Parallel  TimeDomain=Discrete-time  UseExternalTs=off  SampleTime=-1  IntegratorMethod=Forward Euler  FilterMethod=Forward Euler  ControllerParametersSource=internal  P=0.245018327394247  I=1  UseKiTs=off  D=18.2758094977982  UseExternalDerivativeSource=off  N=17.9496179817315  UseFilter=on  TunerSelectOption=Transfer Function Based (PID Tuner App)  InitialConditionSource=internal  InitialConditionForIntegrator=0  InitialConditionForFilter=0  DifferentiatorICPrevScaledInput=0  ExternalReset=none  TrackingMode=off  Kt=1  LimitOutput=off  SatLimitsSource=internal  UpperSaturationLimit=inf  LowerSaturationLimit=-inf  LinearizeAsGain=on  AntiWindupMode=none  Kb=1  LimitIntegrator=off  UpperIntegratorSaturationLimit=inf  LowerIntegratorSaturationLimit=-inf  POutMin=[]  POutMax=[]  IOutMin=[]  IOutMax=[]  DOutMin=[]  DOutMax=[]  NOutMin=[]  NOutMax=[]  SumOutMin=[]  SumOutMax=[]  SaturationOutMin=[]  SaturationOutMax=[]  PParamMin=[]  PParamMax=[]  IParamMin=[]  IParamMax=[]  DParamMin=[]  DParamMax=[]  NParamMin=[]  NParamMax=[]  KbParamMin=[]  KbParamMax=[]  KtParamMin=[]  KtParamMax=[]  KbOutMin=[]  KbOutMax=[]  KtOutMin=[]  KtOutMax=[]  IntegratorOutMin=[]  IntegratorOutMax=[]  FilterOutMin=[]  FilterOutMax=[]  SumI1OutMin=[]  SumI1OutMax=[]  SumI2OutMin=[]  SumI2OutMax=[]  SumI3OutMin=[]  SumI3OutMax=[]  SumI4OutMin=[]  SumI4OutMax=[]  SumDOutMin=[]  SumDOutMax=[]  DifferentiatorOutMin=[]  DifferentiatorOutMax=[]  FilterDiffOutCoefMin=[]  FilterDiffOutCoefMax=[]  ReciprocalOutMin=[]  ReciprocalOutMax=[]  SumDenOutMin=[]  SumDenOutMax=[]  SumNumOutMin=[]  SumNumOutMax=[]  DivideOutMin=[]  DivideOutMax=[]  UdiffTsProdOutMin=[]  UdiffTsProdOutMax=[]  NTsProdOutMin=[]  NTsProdOutMax=[]  UintegralTsProdOutMin=[]  UintegralTsProdOutMax=[]  UngainTsProdOutMin=[]  UngainTsProdOutMax=[]  ClampingZeroOutDataTypeStr=Inherit: Inherit via back propagation  ClampingZeroOutMin=[]  ClampingZeroOutMax=[]  FilterDenConstantOutDataTypeStr=Inherit: Inherit via back propagation  FilterDenConstantOutMin=[]  FilterDenConstantOutMax=[]  PCopyOutDataTypeStr=Inherit: Inherit via back propagation  PCopyOutMin=[]  PCopyOutMax=[]  NCopyOutDataTypeStr=Inherit: Inherit via back propagation  NCopyOutMin=[]  NCopyOutMax=[]  IntegratorContinuousStateAttributes=''  IntegratorStateMustResolveToSignalObject=off  IntegratorRTWStateStorageClass=Auto  FilterContinuousStateAttributes=''  FilterStateMustResolveToSignalObject=off  FilterRTWStateStorageClass=Auto  ParallelPVariant=InternalParameters  IdealPVariant=Disabled  IVariant=Disabled  DVariant=InternalParameters  IntegratorVariant=Disabled  SatVariant=Disabled  AWVariant=Disabled  PCopyVariant=Disabled  TRVariant=Disabled  FdbkBlocksVariant=Forward  IdealPFdbkVariant=Disabled  SatFdbkVariant=Disabled  DerivativeFilterVariant=ForwardEulerFilter  NVariant=InternalParameters  NCopyVariant=Disabled  FilterICVariant=InternalICsFilter  IntegratorICVariant=Disabled  ExternalResetVariant=Disabled  TRSumVariant=Passthrough  SumFdbkVariant=Disabled  SumVariant=Sum_PD  TsampFilterVariant=InternalTs  TsampNgainVariant=Passthrough  TsampIntegralVariant=Disabled_SignalSpec  ExternalSaturationOutDataTypeStr=Inherit: Same as second input  DerivativeSourceVariant=ErrorSignal  PreIntVariant=InternalPreInt
  PID Controller2 : slpidlib/PID Controller  Controller=PD  Form=Parallel  TimeDomain=Discrete-time  UseExternalTs=off  SampleTime=-1  IntegratorMethod=Forward Euler  FilterMethod=Forward Euler  ControllerParametersSource=internal  P=0.245018327394247  I=1  UseKiTs=off  D=18.2758094977982  UseExternalDerivativeSource=off  N=17.9496179817315  UseFilter=on  TunerSelectOption=Transfer Function Based (PID Tuner App)  InitialConditionSource=internal  InitialConditionForIntegrator=0  InitialConditionForFilter=0  DifferentiatorICPrevScaledInput=0  ExternalReset=none  TrackingMode=off  Kt=1  LimitOutput=off  SatLimitsSource=internal  UpperSaturationLimit=inf  LowerSaturationLimit=-inf  LinearizeAsGain=on  AntiWindupMode=none  Kb=1  LimitIntegrator=off  UpperIntegratorSaturationLimit=inf  LowerIntegratorSaturationLimit=-inf  POutMin=[]  POutMax=[]  IOutMin=[]  IOutMax=[]  DOutMin=[]  DOutMax=[]  NOutMin=[]  NOutMax=[]  SumOutMin=[]  SumOutMax=[]  SaturationOutMin=[]  SaturationOutMax=[]  PParamMin=[]  PParamMax=[]  IParamMin=[]  IParamMax=[]  DParamMin=[]  DParamMax=[]  NParamMin=[]  NParamMax=[]  KbParamMin=[]  KbParamMax=[]  KtParamMin=[]  KtParamMax=[]  KbOutMin=[]  KbOutMax=[]  KtOutMin=[]  KtOutMax=[]  IntegratorOutMin=[]  IntegratorOutMax=[]  FilterOutMin=[]  FilterOutMax=[]  SumI1OutMin=[]  SumI1OutMax=[]  SumI2OutMin=[]  SumI2OutMax=[]  SumI3OutMin=[]  SumI3OutMax=[]  SumI4OutMin=[]  SumI4OutMax=[]  SumDOutMin=[]  SumDOutMax=[]  DifferentiatorOutMin=[]  DifferentiatorOutMax=[]  FilterDiffOutCoefMin=[]  FilterDiffOutCoefMax=[]  ReciprocalOutMin=[]  ReciprocalOutMax=[]  SumDenOutMin=[]  SumDenOutMax=[]  SumNumOutMin=[]  SumNumOutMax=[]  DivideOutMin=[]  DivideOutMax=[]  UdiffTsProdOutMin=[]  UdiffTsProdOutMax=[]  NTsProdOutMin=[]  NTsProdOutMax=[]  UintegralTsProdOutMin=[]  UintegralTsProdOutMax=[]  UngainTsProdOutMin=[]  UngainTsProdOutMax=[]  ClampingZeroOutDataTypeStr=Inherit: Inherit via back propagation  ClampingZeroOutMin=[]  ClampingZeroOutMax=[]  FilterDenConstantOutDataTypeStr=Inherit: Inherit via back propagation  FilterDenConstantOutMin=[]  FilterDenConstantOutMax=[]  PCopyOutDataTypeStr=Inherit: Inherit via back propagation  PCopyOutMin=[]  PCopyOutMax=[]  NCopyOutDataTypeStr=Inherit: Inherit via back propagation  NCopyOutMin=[]  NCopyOutMax=[]  IntegratorContinuousStateAttributes=''  IntegratorStateMustResolveToSignalObject=off  IntegratorRTWStateStorageClass=Auto  FilterContinuousStateAttributes=''  FilterStateMustResolveToSignalObject=off  FilterRTWStateStorageClass=Auto  ParallelPVariant=InternalParameters  IdealPVariant=Disabled  IVariant=Disabled  DVariant=InternalParameters  IntegratorVariant=Disabled  SatVariant=Disabled  AWVariant=Disabled  PCopyVariant=Disabled  TRVariant=Disabled  FdbkBlocksVariant=Forward  IdealPFdbkVariant=Disabled  SatFdbkVariant=Disabled  DerivativeFilterVariant=ForwardEulerFilter  NVariant=InternalParameters  NCopyVariant=Disabled  FilterICVariant=InternalICsFilter  IntegratorICVariant=Disabled  ExternalResetVariant=Disabled  TRSumVariant=Passthrough  SumFdbkVariant=Disabled  SumVariant=Sum_PD  TsampFilterVariant=InternalTs  TsampNgainVariant=Passthrough  TsampIntegralVariant=Disabled_SignalSpec  ExternalSaturationOutDataTypeStr=Inherit: Same as second input  DerivativeSourceVariant=ErrorSignal  PreIntVariant=InternalPreInt
  Signal Generator1 : SignalGenerator  Frequency=2*pi/60  Units=rad/sec
  Signal Generator2 : SignalGenerator  Amplitude=0.01  Frequency=2*pi/60  Units=rad/sec
  Sum : Sum  Inputs=-+|
  Sum1 : Sum  Inputs=-+|
  Sum2 : Sum  Inputs=|+-
  Sum3 : Sum  Inputs=|++
  Sum4 : Sum  Inputs=|++
  XY Graph : Record  FileSettingsInternal="{\"entries\":[{\"content\":{\"excelSettings\":{\"content\":{},\"type\":\"Streamout.ExcelSettings\"}},\"type\":\"Streamout.FileSettingStorage\",\"uuid\":\"\"}],\"packageUris\":[\"http:\\/\\/schema.mathworks.com\\/mf0\\/streamout_blocks\\/R2020a\"],\"version\":\"1.0\"}"  Layout=[1 1]  SignalsInternal="{\"entries\":[{\"content\":{},\"type\":\"RecordBlkView.InputSignals\",\"uuid\":\"\"}],\"packageUris\":[\"http:\\/\\/schema.mathworks.com\\/mf0\\/streamout_blocks\\/R2020a\"],\"version\":\"1.0\"}"  VisualizationBindings="{\"xyplotplugin\":{\"info\":[{\"series\":[],\"subplotID\":1}]}}"  CompatibilityTag=XY
  u : Outport
  x : Outport  Port=2
  wires:
  Discrete-Time Integrator4/1 -> Discrete-Time Integrator5/1, Mux1/1
  Discrete-Time Integrator3/1 -> Discrete-Time Integrator2/1, Mux1/2
  Discrete-Time Integrator/1 -> Discrete-Time Integrator1/1, Mux1/3
  Discrete-Time Integrator1/1 -> Sum2/2, Mux/3
  Discrete-Time Integrator2/1 -> Mux/2, Sum1/1
  Discrete-Time Integrator5/1 -> Mux/1, Sum/1
  PID Controller2/1 -> Gain5/1
  PID Controller1/1 -> Gain4/1
  PID Controller/1 -> Gain3/1
  Mux/1 -> Mux2/1
  Mux1/1 -> Mux2/2
  Mux2/1 -> XY Graph/2, x/1
  Gain/1 -> Discrete-Time Integrator4/1
  Gain1/1 -> Discrete-Time Integrator3/1
  Gain2/1 -> Discrete-Time Integrator/1
  Mux3/1 -> u/1
  Sum/1 -> PID Controller2/1
  Sum2/1 -> PID Controller/1
  Sum1/1 -> PID Controller1/1
  Sum4/1 -> Sum1/2
  Constant/1 -> Sum3/2
  Signal Generator1/1 -> Discrete Derivative/1, Sum3/1
  Constant1/1 -> Sum4/2
  Discrete Derivative/1 -> Sum4/1
  Signal Generator2/1 -> Sum2/1
  Sum3/1 -> Sum/2
  Gain3/1 -> Mux3/3, Gain2/1
  Gain4/1 -> Gain1/1, Mux3/2
  Gain5/1 -> Gain/1, Mux3/1

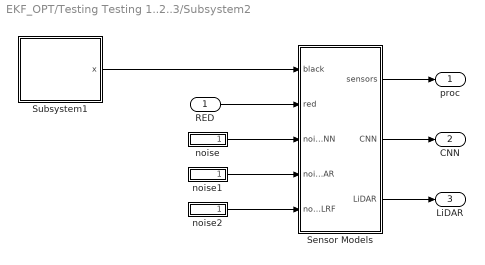
== system EKF_OPT/Testing Testing 1..2..3/Subsystem2 ==
  RED : Inport
  Sensor Models : MATLAB Function  TreatAsAtomicUnit=on
  Subsystem1 : Subsystem
  noise : Subsystem
  noise1 : Subsystem
  noise2 : Subsystem
  proc : Outport
  CNN : Outport  Port=2
  LiDAR : Outport  Port=3
  wires:
  Sensor Models/1(sensors) -> proc/1
  RED/1 -> Sensor Models/2(red)
  Subsystem1/1(x) -> Sensor Models/1(black)
  noise1/1(Out1) -> Sensor Models/4(noiseLiDAR)
  noise/1(Out1) -> Sensor Models/3(noiseCNN)
  noise2/1(Out1) -> Sensor Models/5(noiseLRF)
  Sensor Models/2(CNN) -> CNN/1
  Sensor Models/3(LiDAR) -> LiDAR/1
